simulink model "Fault5StepsSimple"  (R2025a)
settings: Solver=VariableStepAuto  StartTime=0.0  StopTime=10.0  RelTol=1e-3
libraries: simulink x2
settings Model: Creator=mahij  LastModifiedBy=mahij

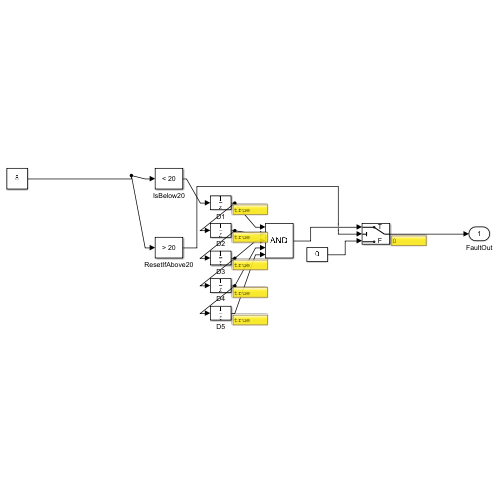
[thumbnail: Simulink's stored preview of the top-level diagram]
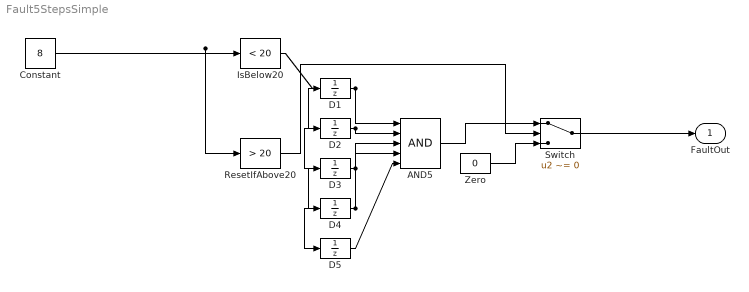
== system Fault5StepsSimple ==
  AND5 : Logic  Inputs=5  AllPortsSameDT=off  OutDataTypeStr=boolean
  Constant : Constant  Value=8
  D{1..5} (5 alike) : UnitDelay  SampleTime=-1  HasFrameUpgradeWarning=on
  IsBelow20 : simulink/Logic and Bit Operations/Compare To Constant  relop=<  const=20  OutDataTypeStr=boolean
  ResetIfAbove20 : simulink/Logic and Bit Operations/Compare To Constant  relop=>  const=20  OutDataTypeStr=boolean
  Switch : Switch  Criteria=u2 ~= 0  Threshold=0.5  SaturateOnIntegerOverflow=off  InputSameDT=off
  Zero : Constant  Value=0
  FaultOut : Outport
  wires:
  Constant/1 -> IsBelow20/1, ResetIfAbove20/1
  IsBelow20/1 -> D1/1
  D1/1 -> D2/1, AND5/1
  D2/1 -> D3/1, AND5/2
  D3/1 -> D4/1, AND5/3
  D4/1 -> D5/1, AND5/4
  D5/1 -> AND5/5
  AND5/1 -> Switch/1
  ResetIfAbove20/1 -> Switch/2
  Zero/1 -> Switch/3
  Switch/1 -> FaultOut/1
